simulink model "Angle_from_sensor_models"  (Simulink 8.3)
settings: Solver=ode3  SolverMode=SingleTasking  StartTime=0.0  StopTime=inf  RelTol=1e-3
settings Model: Creator=Abdou  LastModifiedBy=Abdou  CovMetricSettings=dwe  CovHtmlReporting=off  covSaveCumulativeToWorkspaceVar=off  CovSaveSingleToWorkspaceVar=off  CovExternalEMLEnable=on  CovSFcnEnable=on  ExtModeTrigDuration=2
settings DataIOCC: LimitDataPoints=off  SaveFormat=StructureWithTime  SignalLoggingSaveFormat=Dataset  ReturnWorkspaceOutputs=on
settings OptimizationCC: EnhancedBackFolding=on  PassReuseOutputArgsAs=Individual arguments  ZeroExternalMemoryAtStartup=off  ZeroInternalMemoryAtStartup=off  OptimizeModelRefInitCode=on  MaxStackSize=64
settings DebuggingCC: UnderspecifiedInitializationDetection=Simplified  MergeDetectMultiDrivingBlocksExec=error  SolverPrmCheckMsg=none  ParameterTunabilityLossMsg=error  FrameProcessingCompatibilityMsg=error  StateNameClashWarn=none  SFUnexpectedBacktrackingDiag=error  SFNoUnconditionalDefaultTransitionDiag=error
settings HardwareCC: ProdBitPerInt=16  ProdBitPerPointer=16  ProdIntDivRoundTo=Zero  ProdEndianess=LittleEndian  ProdWordSize=8  ProdHWDeviceType=Atmel->AVR
settings ModelReferenceCC: PropagateSignalLabelsOutOfModel=on
settings SFSimCC: SimUseLocalCustomCode=on
settings RTWCC: Description=Embedded Coder  SystemTargetFile=ert.tlc  TLCOptions=-aInlineSetEventsForThisBaseRateFcn=TLC_FALSE -aSuppressMultiTaskScheduler=TLC_FALSE -aRateBasedStepFcn=1  TemplateMakefile=ert_default_tmf  RTWUseLocalCustomCode=on  Toolchain=Arduino AVR
settings MATStruct: className=codertarget.tools.BuildHook  argsTopModelOnly=[]  excludedModels=[]  includeReferencedModels=on  includeTopModel=on  enabled=on  UseCoderTarget=[1.0]  TargetHardware=Arduino Uno  RTOS=Baremetal  Scheduler_interrupt_source=[0.0]  DataVersion=2016.02  IPAddress=codertarget.arduinobase.registry.getLoopbackIP;  Port=17725  Verbose=[0.0]  Baudrate=codertarget.arduinobase.registry.getBaudRate  COMPort=codertarget.arduinobase.internal.getExternalModeMexArgs('Serial')  Configuration=Serial  COMPortBaud=921600  HostInterface=Simulink  signalBufferSize=[250.0]  Running=on  BuildAction=Build, load and run  DisableParallelBuild=[0.0]  ForceBuildStaticLibrary=[1.0]  Set_host_COM_port=Manually  COM_port_number=6  Enable_SimulinkIO=[1.0]  Enable_overrun_detection=[0.0]  Digital_output_to_set_on_overrun=13  Analog_input_reference_voltage=[0.0]  Serial0_baud_rate=9600  I2C0BusSpeedHz=100000  SPI_clock_out_frequency=4000  SPI_mode=Mode 0 - Clock Polarity 0, Clock Phase 0  SPI_bitorder=MSB first  SDSlaveSelect=[4.0]  CANChipSelect=[9.0]  Disable_DHCP_Ethernet=[0.0]  Local_ip_address=192.168.0.20  Local_mac_address=DE:AD:BE:EF:FE:ED  Wifi_Hardware=WiFi shield  Disable_DHCP_Wifi=[0.0]  Wifi_ip_address=192.168.1.20  Wifi_SSID=yourNetwork  Set_Wifi_Encryption=None  Wifi_WEP_key=D0D0DEADF00DABBADEAFBEADED  Wifi_WEP_key_index=0  Wifi_WPA_password=secretPassword  Wifi_ESP8266_HW_serial_port=Serial 0  Enable_CustomServer=0  IP_address=184.106.153.149  CANBusSpeed=500  CANOscillatorFrequency=16  InterruptPin=[2.0]  AllowAllFilter=[0.0]  Buffer0IDType=Normal  AcceptanceMask0_Nor=0  AcceptanceFilter0_Nor=255  AcceptanceFilter1_Nor=255  AcceptanceMask0_Ext=0  AcceptanceFilter0_Ext=255  AcceptanceFilter1_Ext=255  Buffer1IDType=Normal  AcceptanceMask1_Nor=0  AcceptanceFilter2_Nor=255  AcceptanceFilter3_Nor=255  AcceptanceFilter4_Nor=255  AcceptanceFilter5_Nor=255  AcceptanceMask1_Ext=0  AcceptanceFilter2_Ext=255  AcceptanceFilter3_Ext=255  AcceptanceFilter4_Ext=255  AcceptanceFilter5_Ext=255  Modbus_comms=RS485  Modbus_mode=Master  Modbus_slaveID=1  Modbus_configCoil=1  Modbus_CoilAddr=0  Modbus_CoilNum=1  Modbus_configInput=1  Modbus_InputAddr=0  Modbus_InputNum=1  Modbus_configHoldingReg=1  Modbus_HoldingRegAddr=0  Modbus_HoldingRegNum=1  Modbus_configInputReg=1  Modbus_InputRegAddr=0  Modbus_InputRegNum=1  Modbus_MasterTimeout=100  RS485_serial=Serial 0  RS485_baud=9600  RS485_Config=SERIAL_8N1  RS485_DEPin=8  RS485_REPin=9
settings CodeAppCC: ForceParamTrailComments=on  IgnoreCustomStorageClasses=off  OperatorAnnotations=on  SimulinkDataObjDesc=on  SFDataObjDesc=on  InsertBlockDesc=on
settings ERTTargetCC: SupportContinuousTime=on  SupportVariableSizeSignals=on  ExtMode=on  ExtModeStaticAllocSize=250  ExtModeMexArgs='127.0.0.1' 0 17725

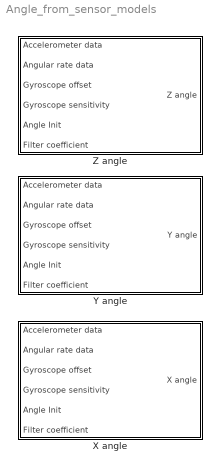
== system Angle_from_sensor_models ==
  X angle : Subsystem
  Y angle : Subsystem
  Z angle : Subsystem

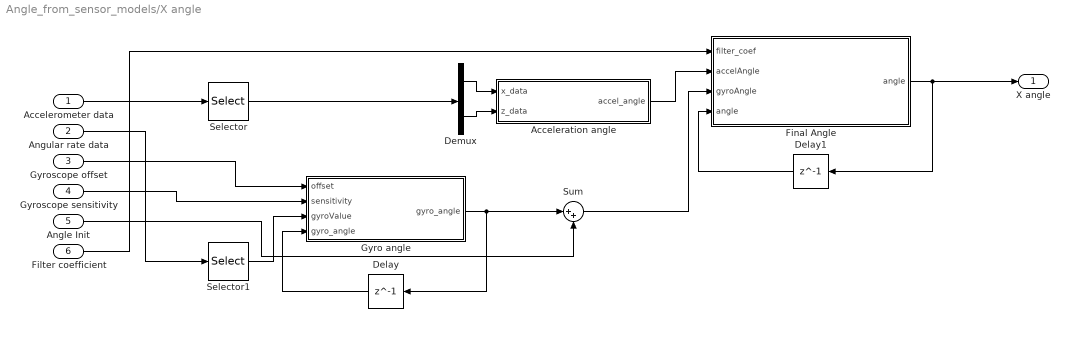
== system Angle_from_sensor_models/X angle ==
  Accelerometer data : Inport
  Angular rate data : Inport  Port=2
  Gyroscope offset : Inport  Port=3
  Gyroscope sensitivity : Inport  Port=4
  Angle Init : Inport  Port=5
  Filter coefficient : Inport  Port=6
  Acceleration angle : MATLAB Function  TreatAsAtomicUnit=on
      settings: PermitHierarchicalResolution=ParametersOnly
  Delay : Delay  DelayLength=1  InitialCondition=0
  Delay1 : Delay  DelayLength=1  InitialCondition=0
  Demux : Demux  Outputs=2
  Final Angle : MATLAB Function  TreatAsAtomicUnit=on
      settings: PermitHierarchicalResolution=ParametersOnly
  Gyro angle : MATLAB Function  TreatAsAtomicUnit=on
      settings: PermitHierarchicalResolution=ParametersOnly
  Selector : Selector  InputPortWidth=3  IndexOptions=Index vector (dialog)  Indices=[2 3]  OutputSizes=1
  Selector1 : Selector  InputPortWidth=3  IndexOptions=Index vector (dialog)  Indices=1  OutputSizes=1
  Sum : Sum  Inputs=|++
  X angle : Outport
  wires:
  Demux/1 -> Acceleration angle/1(x_data)
  Sum/1 -> Final Angle/3(gyroAngle)
  Delay/1 -> Gyro angle/4("gyro_angle ")
  Angle Init/1 -> Sum/2
  Demux/2 -> Acceleration angle/2(z_data)
  Gyro angle/1(gyro_angle) -> Sum/1, Delay/1
  Selector1/1 -> Gyro angle/3(gyroValue)
  Final Angle/1(angle) -> X angle/1, Delay1/1
  Filter coefficient/1 -> Final Angle/1(filter_coef)
  Selector/1 -> Demux/1
  Acceleration angle/1(accel_angle) -> Final Angle/2(accelAngle)
  Delay1/1 -> Final Angle/4("angle ")
  Gyroscope sensitivity/1 -> Gyro angle/2(sensitivity)
  Accelerometer data/1 -> Selector/1
  Angular rate data/1 -> Selector1/1
  Gyroscope offset/1 -> Gyro angle/1(offset)

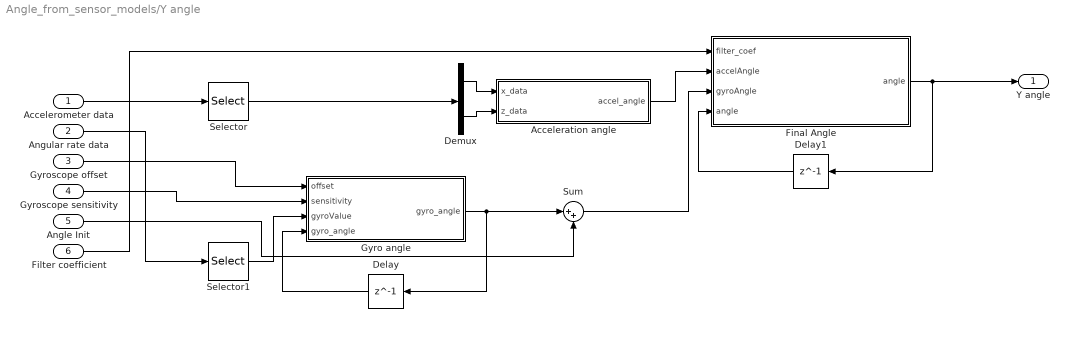
== system Angle_from_sensor_models/Y angle ==
  Accelerometer data : Inport
  Angular rate data : Inport  Port=2
  Gyroscope offset : Inport  Port=3
  Gyroscope sensitivity : Inport  Port=4
  Angle Init : Inport  Port=5
  Filter coefficient : Inport  Port=6
  Acceleration angle : MATLAB Function  TreatAsAtomicUnit=on
      settings: PermitHierarchicalResolution=ParametersOnly
  Delay : Delay  DelayLength=1  InitialCondition=0
  Delay1 : Delay  DelayLength=1  InitialCondition=0
  Demux : Demux  Outputs=2
  Final Angle : MATLAB Function  TreatAsAtomicUnit=on
      settings: PermitHierarchicalResolution=ParametersOnly
  Gyro angle : MATLAB Function  TreatAsAtomicUnit=on
      settings: PermitHierarchicalResolution=ParametersOnly
  Selector : Selector  InputPortWidth=3  IndexOptions=Index vector (dialog)  Indices=[1 3]  OutputSizes=1
  Selector1 : Selector  InputPortWidth=3  IndexOptions=Index vector (dialog)  Indices=2  OutputSizes=1
  Sum : Sum  Inputs=|++
  Y angle : Outport
  wires:
  Demux/1 -> Acceleration angle/1(x_data)
  Sum/1 -> Final Angle/3(gyroAngle)
  Delay/1 -> Gyro angle/4("gyro_angle ")
  Angle Init/1 -> Sum/2
  Demux/2 -> Acceleration angle/2(z_data)
  Gyro angle/1(gyro_angle) -> Sum/1, Delay/1
  Selector1/1 -> Gyro angle/3(gyroValue)
  Final Angle/1(angle) -> Y angle/1, Delay1/1
  Filter coefficient/1 -> Final Angle/1(filter_coef)
  Selector/1 -> Demux/1
  Acceleration angle/1(accel_angle) -> Final Angle/2(accelAngle)
  Delay1/1 -> Final Angle/4("angle ")
  Gyroscope sensitivity/1 -> Gyro angle/2(sensitivity)
  Accelerometer data/1 -> Selector/1
  Angular rate data/1 -> Selector1/1
  Gyroscope offset/1 -> Gyro angle/1(offset)

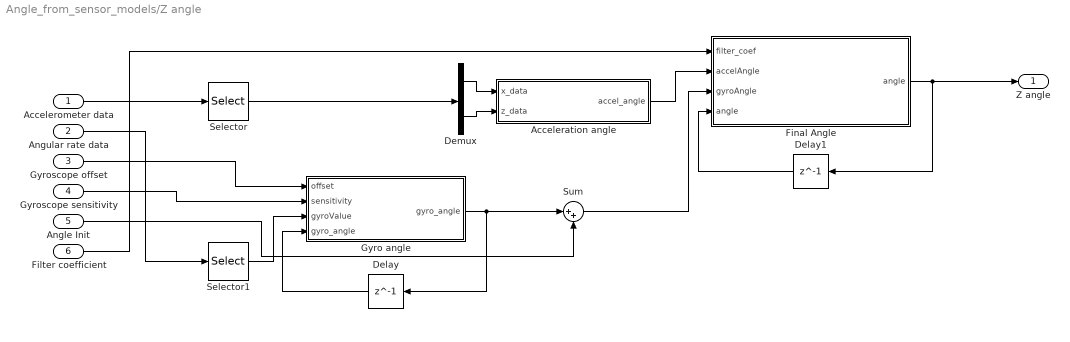
== system Angle_from_sensor_models/Z angle ==
  Accelerometer data : Inport
  Angular rate data : Inport  Port=2
  Gyroscope offset : Inport  Port=3
  Gyroscope sensitivity : Inport  Port=4
  Angle Init : Inport  Port=5
  Filter coefficient : Inport  Port=6
  Acceleration angle : MATLAB Function  TreatAsAtomicUnit=on
      settings: PermitHierarchicalResolution=ParametersOnly
  Delay : Delay  DelayLength=1  InitialCondition=0
  Delay1 : Delay  DelayLength=1  InitialCondition=0
  Demux : Demux  Outputs=2
  Final Angle : MATLAB Function  TreatAsAtomicUnit=on
      settings: PermitHierarchicalResolution=ParametersOnly
  Gyro angle : MATLAB Function  TreatAsAtomicUnit=on
      settings: PermitHierarchicalResolution=ParametersOnly
  Selector : Selector  InputPortWidth=3  IndexOptions=Index vector (dialog)  Indices=[1 2]  OutputSizes=1
  Selector1 : Selector  InputPortWidth=3  IndexOptions=Index vector (dialog)  Indices=3  OutputSizes=1
  Sum : Sum  Inputs=|++
  Z angle : Outport
  wires:
  Demux/1 -> Acceleration angle/1(x_data)
  Sum/1 -> Final Angle/3(gyroAngle)
  Delay/1 -> Gyro angle/4("gyro_angle ")
  Angle Init/1 -> Sum/2
  Demux/2 -> Acceleration angle/2(z_data)
  Gyro angle/1(gyro_angle) -> Sum/1, Delay/1
  Selector1/1 -> Gyro angle/3(gyroValue)
  Final Angle/1(angle) -> Z angle/1, Delay1/1
  Filter coefficient/1 -> Final Angle/1(filter_coef)
  Selector/1 -> Demux/1
  Acceleration angle/1(accel_angle) -> Final Angle/2(accelAngle)
  Delay1/1 -> Final Angle/4("angle ")
  Gyroscope sensitivity/1 -> Gyro angle/2(sensitivity)
  Accelerometer data/1 -> Selector/1
  Angular rate data/1 -> Selector1/1
  Gyroscope offset/1 -> Gyro angle/1(offset)

== matlab function Z angle/Final Angle ==
  data: filter_coef input double; accelAngle input double; gyroAngle input double; angle output double; angle input double
function angle = Complimentary_filter(filter_coef,accelAngle,gyroAngle,angle)
    angle = filter_coef * (angle + gyroAngle / 100 ) + (1 - filter_coef) * accelAngle;

== matlab function Z angle/Gyro angle ==
  data: offset input double; sensitivity input double; gyroValue input double; gyro_angle output double; gyro_angle input double
function gyro_angle = Gyro_angle(offset,sensitivity,gyroValue,gyro_angle)
    gyroRate = (gyroValue - offset) * sensitivity;
    gyro_angle = gyro_angle - gyroRate / 100.0;

== matlab function Z angle/Acceleration angle ==
  data: x_data input double; z_data input double; accel_angle output double
function accel_angle = Accel_angle(x_data,z_data)
    accel_angle = atan2(x_data,z_data) * 180/pi ;

== matlab function Y angle/Acceleration angle ==
  data: x_data input double; z_data input double; accel_angle output double
function accel_angle = Accel_angle(x_data,z_data)
    accel_angle = atan2(x_data,z_data) * 180/pi ;

== matlab function Y angle/Final Angle ==
  data: filter_coef input double; accelAngle input double; gyroAngle input double; angle output double; angle input double
function angle = Complimentary_filter(filter_coef,accelAngle,gyroAngle,angle)
    angle = filter_coef * (angle + gyroAngle / 100 ) + (1 - filter_coef) * accelAngle;

== matlab function Y angle/Gyro angle ==
  data: offset input double; sensitivity input double; gyroValue input double; gyro_angle output double; gyro_angle input double
function gyro_angle = Gyro_angle(offset,sensitivity,gyroValue,gyro_angle)
    gyroRate = (gyroValue - offset) * sensitivity;
    gyro_angle = gyro_angle - gyroRate / 100.0;

== matlab function X angle/Acceleration angle ==
  data: x_data input double; z_data input double; accel_angle output double
function accel_angle = Accel_angle(x_data,z_data)
    accel_angle = atan2(x_data,z_data) * 180/pi ;

== matlab function X angle/Final Angle ==
  data: filter_coef input double; accelAngle input double; gyroAngle input double; angle output double; angle input double
function angle = Complimentary_filter(filter_coef,accelAngle,gyroAngle,angle)
    angle = filter_coef * (angle + gyroAngle / 100 ) + (1 - filter_coef) * accelAngle;

== matlab function X angle/Gyro angle ==
  data: offset input double; sensitivity input double; gyroValue input double; gyro_angle output double; gyro_angle input double
function gyro_angle = Gyro_angle(offset,sensitivity,gyroValue,gyro_angle)
    gyroRate = (gyroValue - offset) * sensitivity;
    gyro_angle = gyro_angle - gyroRate / 100.0;
